simulink model "SEIRS_Ruido"  (R2024a)
settings: Solver=VariableStepAuto  StartTime=0.0  StopTime=T  RelTol=1e-3
undefined symbols (not defined in the file or in its folder): var_init
settings Model: Creator=carlo  LastModifiedBy=luism
settings DataIOCC: SaveOutput=off
settings RTWCC: GPUComputeCapability=3.5

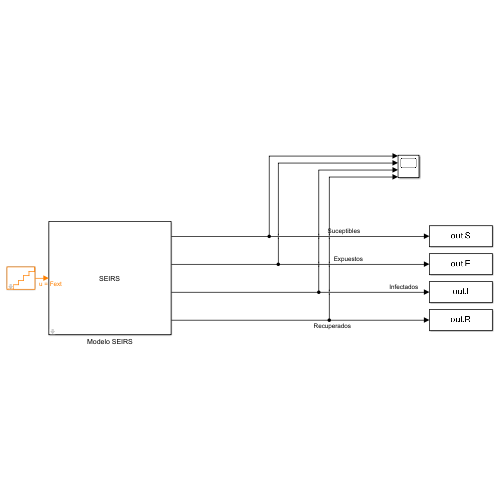
[thumbnail: Simulink's stored preview of the top-level diagram]
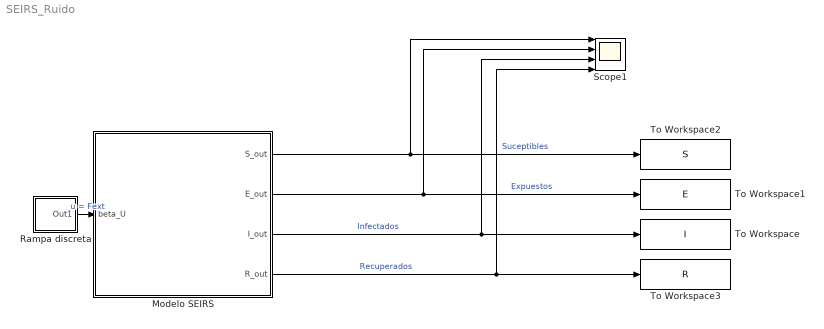
== system SEIRS_Ruido ==
  Modelo SEIRS : Subsystem  mask{B=var_init(1), d=var_init(2), alpha=var_init(3), gamma=var_init(4), beta=var_init(5), nu=var_init(6), ci=[0.1431 0.0092 0.0092 0.8384], Ruido=on}
      mask prompts: ci "[S0 E0 I0 R0]"; Ruido "Incluir ruido al sistema"
      mask Display: disp('SEIRS');
  Rampa discreta : Subsystem  mask(Rampa discreta){x0=0, Ts=2000, du=0.1}
      mask prompts: x0 "Valor inicial"; Ts "Ancho de cada escalón"; du "Alto de cada escalón"
      mask help: Rampa discreta con período de muestreo Ts e incrementos du.
      mask Display: plot([0 1 1 2 2 3 3 4 4 5 5],[0 0 1 1 2 2 3 3 4 4 5])
  Scope1 : Scope  NumInputPorts=4
  To Workspace : ToWorkspace  VariableName=I  SaveFormat=Structure With Time  SampleTime=-1
  To Workspace1 : ToWorkspace  VariableName=E  SaveFormat=Structure With Time  SampleTime=-1
  To Workspace2 : ToWorkspace  VariableName=S  SaveFormat=Structure With Time  SampleTime=-1
  To Workspace3 : ToWorkspace  VariableName=R  SaveFormat=Structure With Time  SampleTime=-1
  wires:
  Modelo SEIRS/3("I_out ") -> To Workspace/1, Scope1/3  "Infectados"
  Modelo SEIRS/1(S_out) -> To Workspace2/1, Scope1/1  "Suceptibles"
  Modelo SEIRS/4(R_out) -> To Workspace3/1, Scope1/4  "Recuperados"
  Modelo SEIRS/2(E_out) -> To Workspace1/1, Scope1/2  "Expuestos"
  Rampa discreta/1(Out1) -> Modelo SEIRS/1(beta_U)  "u = Fext"

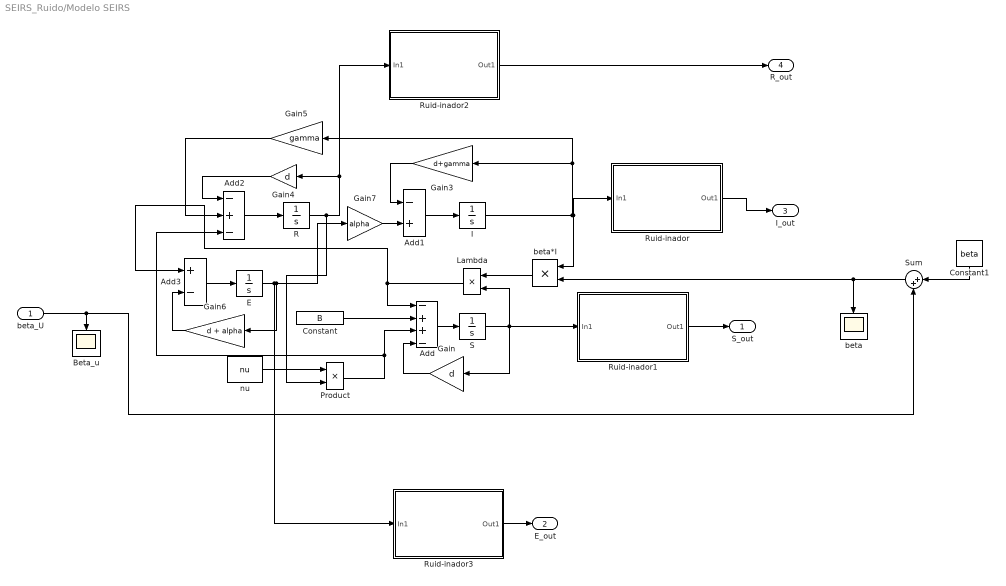
== system SEIRS_Ruido/Modelo SEIRS ==
  beta_U : Inport
  Add : Sum  Inputs=-++-
  Add1 : Sum  Inputs=-+
  Add2 : Sum  Inputs=-+-
  Add3 : Sum  Inputs=+-
  Beta_u : Scope
  Constant : Constant  Value=B
  Constant1 : Constant  Value=beta
  E : Integrator  InitialCondition=ci(2)  LimitOutput=on  LowerSaturationLimit=0
  Gain : Gain  Gain=d
  Gain3 : Gain  Gain=d+gamma
  Gain4 : Gain  Gain=d
  Gain5 : Gain  Gain=gamma
  Gain6 : Gain  Gain=d + alpha
  Gain7 : Gain  Gain=alpha
  I : Integrator  InitialCondition=ci(3)  LimitOutput=on  LowerSaturationLimit=0
  Lambda : Product
  Product : Product
  R : Integrator  InitialCondition=ci(4)  LimitOutput=on  LowerSaturationLimit=0
  Ruid-inador : Subsystem
      mask Display: image('ruido_inador.jpeg');
  Ruid-inador1 : Subsystem
      mask Display: image('ruido_inador.jpeg');
  Ruid-inador2 : Subsystem
      mask Display: image('ruido_inador.jpeg');
  Ruid-inador3 : Subsystem
      mask Display: image('ruido_inador.jpeg');
  S : Integrator  InitialCondition=ci(1)  LimitOutput=on  LowerSaturationLimit=0
  Sum : Sum  Inputs=|++
  beta : Scope
  beta*I : Product
  nu : Constant  Value=nu
  S_out : Outport
  E_out : Outport  Port=2
  "I_out " : Outport  Port=3
  R_out : Outport  Port=4
  wires:
  Gain/1 -> Add/4
  Gain4/1 -> Add2/1
  Constant/1 -> Add/2
  I/1 -> Ruid-inador/1(In1), beta*I/1, Gain5/1, Gain3/1
  Lambda/1 -> Add3/1, Add/1
  Add/1 -> S/1
  E/1 -> Gain7/1, Gain6/1, Ruid-inador3/1(In1)
  S/1 -> Ruid-inador1/1(In1), Lambda/2, Gain/1
  Add3/1 -> E/1
  Gain3/1 -> Add1/1
  Gain5/1 -> Add2/2
  Gain6/1 -> Add3/2
  Add1/1 -> I/1
  R/1 -> Ruid-inador2/1(In1), Gain4/1, Product/2
  Add2/1 -> R/1
  Product/1 -> Add2/3, Add/3
  Gain7/1 -> Add1/2
  nu/1 -> Product/1
  beta*I/1 -> Lambda/1
  Sum/1 -> beta*I/2, beta/1
  Constant1/1 -> Sum/1
  beta_U/1 -> Sum/2, Beta_u/1
  Ruid-inador/1(Out1) -> "I_out "/1
  Ruid-inador2/1(Out1) -> R_out/1
  Ruid-inador1/1(Out1) -> S_out/1
  Ruid-inador3/1(Out1) -> E_out/1

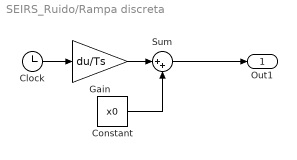
== system SEIRS_Ruido/Rampa discreta ==
  Clock : Clock
      settings: DisableCoverage=on
  Constant : Constant  Value=x0
  Gain : Gain  Gain=du/Ts  SampleTime=Ts
  Sum : Sum  Inputs=|++
  Out1 : Outport
  wires:
  Clock/1 -> Gain/1
  Gain/1 -> Sum/1
  Sum/1 -> Out1/1
  Constant/1 -> Sum/2

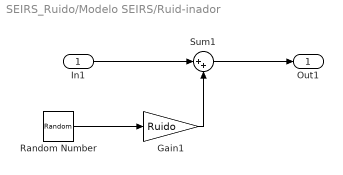
== system SEIRS_Ruido/Modelo SEIRS/Ruid-inador ==
  In1 : Inport
  Gain1 : Gain  Gain=Ruido
  Random Number : RandomNumber  Variance=1e-9  Seed=117  SampleTime=0.1
  Sum1 : Sum  Inputs=|++
  Out1 : Outport
  wires:
  Random Number/1 -> Gain1/1
  Gain1/1 -> Sum1/2
  In1/1 -> Sum1/1
  Sum1/1 -> Out1/1

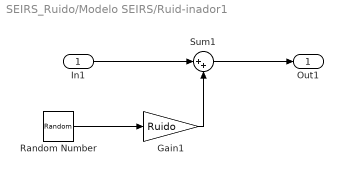
== system SEIRS_Ruido/Modelo SEIRS/Ruid-inador1 ==
  In1 : Inport
  Gain1 : Gain  Gain=Ruido
  Random Number : RandomNumber  Variance=1e-9  Seed=117  SampleTime=0.1
  Sum1 : Sum  Inputs=|++
  Out1 : Outport
  wires:
  Random Number/1 -> Gain1/1
  Gain1/1 -> Sum1/2
  In1/1 -> Sum1/1
  Sum1/1 -> Out1/1

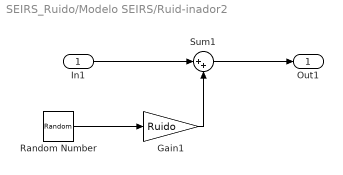
== system SEIRS_Ruido/Modelo SEIRS/Ruid-inador2 ==
  In1 : Inport
  Gain1 : Gain  Gain=Ruido
  Random Number : RandomNumber  Variance=1e-9  Seed=117  SampleTime=0.1
  Sum1 : Sum  Inputs=|++
  Out1 : Outport
  wires:
  Random Number/1 -> Gain1/1
  Gain1/1 -> Sum1/2
  In1/1 -> Sum1/1
  Sum1/1 -> Out1/1

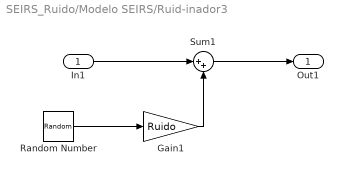
== system SEIRS_Ruido/Modelo SEIRS/Ruid-inador3 ==
  In1 : Inport
  Gain1 : Gain  Gain=Ruido
  Random Number : RandomNumber  Variance=1e-9  Seed=117  SampleTime=0.1
  Sum1 : Sum  Inputs=|++
  Out1 : Outport
  wires:
  Random Number/1 -> Gain1/1
  Gain1/1 -> Sum1/2
  In1/1 -> Sum1/1
  Sum1/1 -> Out1/1
